simulink model "testSampleBeam"  (R2019b)
settings: configuration reference "cset" (kept outside this file)
PreLoadFcn:
  | disp(['Executing PreLoadFcn in ' get_param(gcs,'Name')])
  | 
  | % Path
  | addpath(fullfile('..','mdl'));
  | 
  | % Load configuration
  | load('testsamplebeam_cset');
  | 
  | % Load bus objects
  | load('SonarWorkbenchPublicBusObjects');
StopFcn:
  | disp(['Executing StopFcn in ' get_param(gcs,'Name')])
  | 
  | % Plot beam pattern
  | PlotNEDaxes(0,0,0)
  | Plot3DBP(theta,psi,BP,[],[],gca)
model workspace (MAT data in the model file):
  Ne = 4
  Ntype = 2
undefined symbols (not defined in the file or in its folder): chebwin
settings Model: Creator=tom  LastModifiedBy=tom
settings ConfigSetRef: SourceName=cset  SourceLocation=Base Workspace

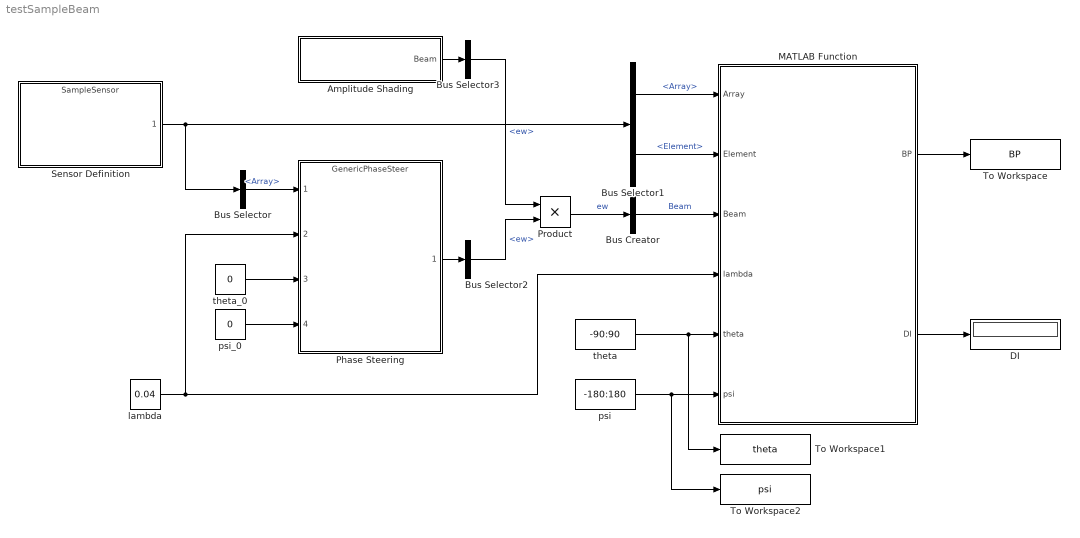
== system testSampleBeam ==
  Amplitude Shading : Subsystem
  Bus Creator : BusCreator  Inputs=1  OutDataTypeStr=Bus: SonarWorkbenchBeamObj
  Bus Selector : BusSelector  OutputSignals=Array
  Bus Selector1 : BusSelector  OutputSignals=Array,Element
  Bus Selector2 : BusSelector  OutputSignals=ew
  Bus Selector3 : BusSelector  OutputSignals=ew
  DI : Display
  MATLAB Function : MATLAB Function  TreatAsAtomicUnit=on
  Phase Steering : ModelReference  ModelNameDialog=GenericPhaseSteer.slx  ModelReferenceVersion=1.20
      mask Display:
      | % Cover port labels
      | patch([0 1 1 0],[0.1 0.1 0.9 0.9],[0.910 0.820 0.322])
      | 
      | % Label ports
      | port_label('input',1,'Array','interpreter','tex')
      | port_label('input',2,'\lambda','interpreter','tex')
      | port_label('input',3,'\theta_0','interpreter','tex')
      | port_label('input',4,'\psi_0','interpreter','tex')
      | port_label('output',1,'Beam','interpreter','tex')
  Product : Product
  Sensor Definition : ModelReference  ModelNameDialog=SampleSensor  ModelReferenceVersion=1.20
  To Workspace : ToWorkspace  VariableName=BP  SampleTime=-1
      settings: MaxDataPoints=1
  To Workspace1 : ToWorkspace  VariableName=theta  SampleTime=-1
      settings: MaxDataPoints=1
  To Workspace2 : ToWorkspace  VariableName=psi  SampleTime=-1
      settings: MaxDataPoints=1
  lambda : Constant  Value=0.04  OutDataTypeStr=double
  psi : Constant  Value=-180:180  OutDataTypeStr=double
  psi_0 : Constant  Value=0  OutDataTypeStr=double
  theta : Constant  Value=-90:90  OutDataTypeStr=double
  theta_0 : Constant  Value=0  OutDataTypeStr=double
  wires:
  theta_0/1 -> Phase Steering/3
  psi_0/1 -> Phase Steering/4
  Bus Selector1/2 -> MATLAB Function/2(Element)  "<Element>"
  lambda/1 -> Phase Steering/2, MATLAB Function/4(lambda)
  theta/1 -> To Workspace1/1, MATLAB Function/5(theta)
  psi/1 -> To Workspace2/1, MATLAB Function/6(psi)
  MATLAB Function/1(BP) -> To Workspace/1
  Sensor Definition/1 -> Bus Selector1/1, Bus Selector/1
  Bus Selector/1 -> Phase Steering/1  "<Array>"
  Bus Selector1/1 -> MATLAB Function/1(Array)  "<Array>"
  Phase Steering/1 -> Bus Selector2/1
  Amplitude Shading/1("Beam ") -> Bus Selector3/1
  Bus Selector3/1 -> Product/1  "<ew>"
  Bus Selector2/1 -> Product/2  "<ew>"
  Product/1 -> Bus Creator/1  "ew"
  Bus Creator/1 -> MATLAB Function/3(Beam)  "Beam"
  MATLAB Function/2(DI) -> DI/1

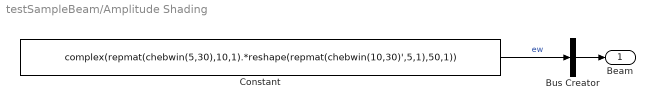
== system testSampleBeam/Amplitude Shading ==
  Bus Creator : BusCreator  Inputs=1  OutDataTypeStr=Bus: SonarWorkbenchBeamObj
  Constant : Constant  Value=complex(repmat(chebwin(5,30),10,1).*reshape(repmat(chebwin(10,30)',5,1),50,1))  VectorParams1D=off  OutDataTypeStr=double
  "Beam " : Outport  OutDataTypeStr=Bus: SonarWorkbenchBeamObj
  wires:
  Constant/1 -> Bus Creator/1  "ew"
  Bus Creator/1 -> "Beam "/1

== matlab function testSampleBeam/MATLAB Function ==
  data: Array input Bus: SonarWorkbenchArrayObj; BP output double size=[181 361]; Element input Bus: SonarWorkbenchElementObj; Beam input Bus: SonarWorkbenchBeamObj; lambda input double size=1; theta input double size=181; psi input double size=361; DI output
function [BP, DI] = EvaluateBeamPattern(Array,Element,Beam,lambda,theta,psi)
%#codegen
Ntheta = length(theta);
Npsi = length(psi);
tmp = BeamPattern(Array,Element,Beam,lambda,theta,psi);
BP = tmp(1:Ntheta,1:Npsi);
DI = CalculateDI(theta,psi,BP);
